simulink model "AngleToPWM"  (R2017b)
settings: Solver=FixedStepDiscrete  StartTime=0.0  StopTime=5000  FixedStep=1  RelTol=1e-3
libraries: hdlsllib x3, simulink x1
settings Model: Creator=chandler.ga  LastModifiedBy=Gavin
settings CodeAppCC: StateflowObjectComments=on

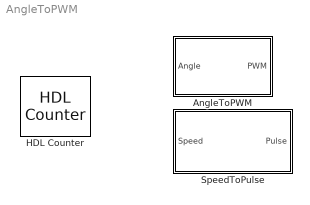
== system AngleToPWM ==
  AngleToPWM : Subsystem
  HDL Counter : hdlsllib/Sources/HDL Counter  CountType=Count limited  CountInit=90  CountStep=1  CountMax=180  CountFromType=Specify  CountFrom=0  CountResetPort=off  CountLoadPort=off  CountEnbPort=on  CountDirPort=on  CountDataType=Unsigned  CountWordLen=8  CountFracLen=0  CountSampTime=1
      settings: SourceProductBaseCode=HD
  SpeedToPulse : Subsystem

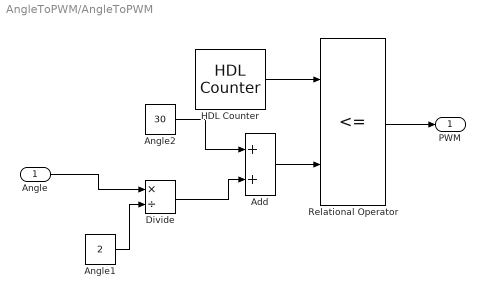
== system AngleToPWM/AngleToPWM ==
  Angle : Inport
  Add : Sum
  Angle1 : Constant  Value=2  OutDataTypeStr=uint8
  Angle2 : Constant  Value=30  OutDataTypeStr=uint8
  Divide : Product  Inputs=*/  SaturateOnIntegerOverflow=on  RndMeth=Zero
  HDL Counter : hdlsllib/Sources/HDL Counter  CountType=Count limited  CountInit=0  CountStep=1  CountMax=1000  CountFromType=Initial value  CountFrom=0  CountResetPort=off  CountLoadPort=off  CountEnbPort=off  CountDirPort=off  CountDataType=Unsigned  CountWordLen=10  CountFracLen=0  CountSampTime=1
      settings: SourceProductBaseCode=HD
  Relational Operator : RelationalOperator  Operator=<=  OutDataTypeStr=boolean  RndMeth=Simplest
  PWM : Outport
  wires:
  Angle/1 -> Divide/1
  Divide/1 -> Add/2
  Relational Operator/1 -> PWM/1
  Add/1 -> Relational Operator/2
  HDL Counter/1 -> Relational Operator/1
  Angle2/1 -> Add/1
  Angle1/1 -> Divide/2

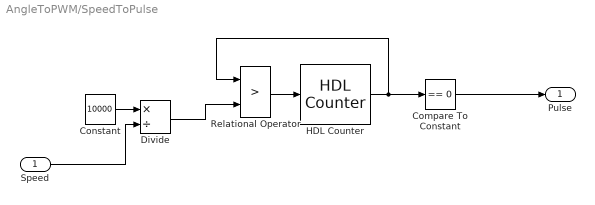
== system AngleToPWM/SpeedToPulse ==
  Speed : Inport  OutDataTypeStr=uint8
  Compare To Constant : simulink/Logic and Bit Operations/Compare To Constant  relop===  const=0  OutDataTypeStr=boolean
  Constant : Constant  Value=10000
  Divide : Product  Inputs=*/  SaturateOnIntegerOverflow=on  RndMeth=Zero
  HDL Counter : hdlsllib/Sources/HDL Counter  CountType=Count limited  CountInit=0  CountStep=1  CountMax=10000  CountFromType=Initial value  CountFrom=0  CountResetPort=on  CountLoadPort=off  CountEnbPort=off  CountDirPort=off  CountDataType=Unsigned  CountWordLen=18  CountFracLen=0  CountSampTime=1
      settings: SourceProductBaseCode=HD
  Relational Operator : RelationalOperator  Operator=>  OutDataTypeStr=boolean  RndMeth=Nearest
  Pulse : Outport
  wires:
  Constant/1 -> Divide/1
  HDL Counter/1 -> Relational Operator/1, Compare To Constant/1
  Divide/1 -> Relational Operator/2
  Speed/1 -> Divide/2
  Compare To Constant/1 -> Pulse/1
  Relational Operator/1 -> HDL Counter/1
